simulink model "car_suspension"  (R2025a)
settings: Solver=VariableStepAuto  StartTime=0.0  StopTime=10.0  RelTol=1e-3
values from neighbouring files (symbols this model uses):
  B = 500    [test.m]
  K1 = 20000    [test.m]
  K2 = 10000    [test.m]
  M1 = 40    [test.m]
  M2 = 250    [test.m]
settings Model: Creator=user  LastModifiedBy=user

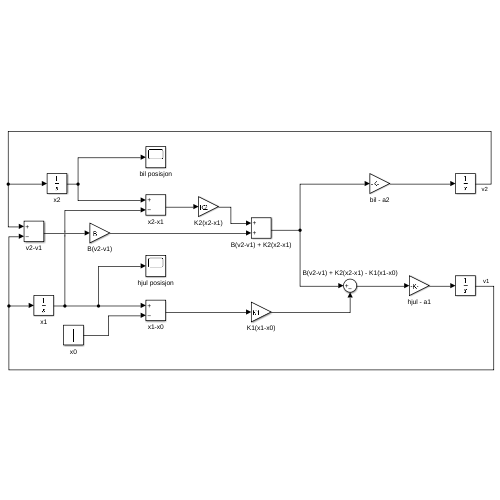
[thumbnail: Simulink's stored preview of the top-level diagram]
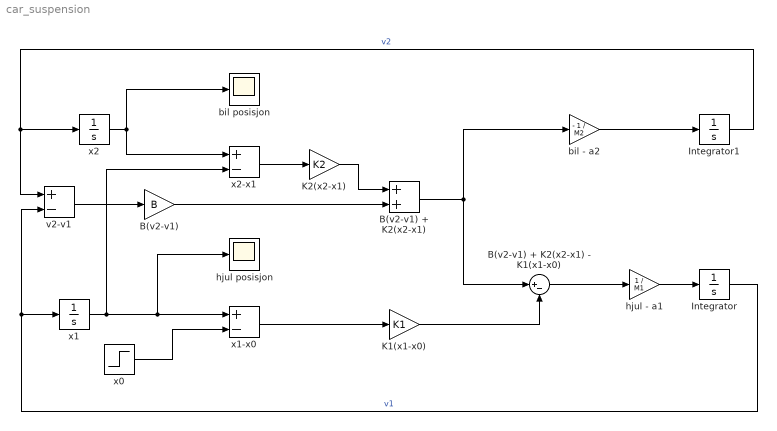
== system car_suspension ==
  B(v2-v1) : Gain  Gain=B
  B(v2-v1) + K2(x2-x1) : Sum
  B(v2-v1) + K2(x2-x1) - K1(x1-x0) : Sum  Inputs=|+-
  Integrator : Integrator
  Integrator1 : Integrator
  K1(x1-x0) : Gain  Gain=K1
  K2(x2-x1) : Gain  Gain=K2
  bil - a2 : Gain  Gain=- 1 / M2
  bil posisjon : Scope
      settings: ActiveDisplayYMinimum=-0.2273283471253493  ActiveDisplayYMaximum=2.0459551241281444
  hjul - a1 : Gain  Gain=1 / M1
  hjul posisjon : Scope
      settings: ActiveDisplayYMinimum=-0.16233251478325914  ActiveDisplayYMaximum=1.4609926330493326
  v2-v1 : Sum  Inputs=+-
  x0 : Step  SampleTime=0
  x1 : Integrator
  x1-x0 : Sum  Inputs=+-
  x2 : Integrator
  x2-x1 : Sum  Inputs=+-
  wires:
  hjul - a1/1 -> Integrator/1
  B(v2-v1) + K2(x2-x1) - K1(x1-x0)/1 -> hjul - a1/1
  Integrator/1 -> x1/1, v2-v1/2  "v1"
  bil - a2/1 -> Integrator1/1
  B(v2-v1) + K2(x2-x1)/1 -> B(v2-v1) + K2(x2-x1) - K1(x1-x0)/1, bil - a2/1
  Integrator1/1 -> x2/1, v2-v1/1  "v2"
  v2-v1/1 -> B(v2-v1)/1
  x2/1 -> bil posisjon/1, x2-x1/1
  x1/1 -> hjul posisjon/1, x1-x0/1, x2-x1/2
  x2-x1/1 -> K2(x2-x1)/1
  K2(x2-x1)/1 -> B(v2-v1) + K2(x2-x1)/1
  B(v2-v1)/1 -> B(v2-v1) + K2(x2-x1)/2
  x0/1 -> x1-x0/2
  x1-x0/1 -> K1(x1-x0)/1
  K1(x1-x0)/1 -> B(v2-v1) + K2(x2-x1) - K1(x1-x0)/2
